simulink model "A1_MIM0_DigiTwin_4cm_JG_BM_2017b"  (R2017b)
settings: Solver=VariableStepAuto  StartTime=0.0  StopTime=tsim  RelTol=1e-3
InitFcn:
  | tsim=1000
  | sg=1;
  | Ts=500 %500% deseado 890-->Ts modelo
  | wn=5.8335/Ts; %2ord
  | wp=4/Ts; %np=1.5; 1ord
  | wt1=8*wn
  | wt=3.5*wn
  | wt3=3.49*wn
  | nf=2.5; %[1.2 1.5 1.75 2 2.5]
  | %Tfp=1/(np*wp)
  | Tf= 1/(nf*wn) % f del filtro;
  | nf3=5
  | Tf3= 1/(nf3*wn)
  | Rpc=0.09 % cold side resistor
  | Rph= 0.6 % hot side resistor
  | Tamb=273.15+15 % ambiental temp
  | Tin=273.15+15 % initial temp of mass
  | %TinA= 284.9405 % internal air Inicial temp
  | %TinAis=  294.0300 % initial Temp Mass insolat
  | %Tp1=283  %ideal temp of  peltier cells
  | %Tp2=Tp1
  | 
  | %Peltier Cells parameter
  | Th=323 % [K]
  | TinH=298
  | TinC=298 %
  | dTmax=75 % 70.5 [K]
  | Vmax= 16.4 % 13.9 [v]
  | Imax= 6.4 % 4  [A]
  | Rth= (dTmax/(Vmax*Imax))*(2*Th/(Th-dTmax)) % Termal Res [K/W]
  | am= Vmax/ Th %  0.054 Seebeck Coef []
  | ReC=Vmax*(Th-dTmax)/(Th*Imax) %range [1.6 1.96 2.5]
  | %Re= 2.3 %2.65   [2.6584  2.9592 3.26]  at 300 K
  | Mc=0.0135; %0.0045  Cool mass [kg]
  | Mh=0.0135; %0.0045
  | Cesp=1262  %1262.2 345
  | %TinL=300
  | %CespL=100 %45
  | %Mload=100%100-0.065 0.001
  | %Rload=1%5.5
  | 
  | 
  | % --Copper & aluminum plate
  | Da= 8960; %2700 [Kg/m^3] density
  | Qs= 390; %970 Specific heat [J/(Kg*K)]
  | Thi =0.00508; % 0.0033 Thickness [m]
  | L = 0.04; %0.03 length [m]
  | L1=0.035;
  | W=0.04; % 0.03 width  [m]
  | W1=0.01; W2=0.03;  W3=0.015;
  | Va= L*W*Thi % 2,97 E-6 [m^3] Dif of Volume
  | M=Da*Va % 0.00801 [kg]  % Al Dif of Mass
  | 
  | %--- Air Properties
  | Thi_air=0.015 % Thickness of air
  | Dair=1.29 % [Kg/m^3] density
  | Vair= L*W*Thi_air % E-6 [m^3] Dif of Volume
  | Mair=Dair*Vair %  [kg]  % Al Dif of Mass
  | 
  | % thermal conductivity [W/(m*K)]
  | K=401; %200  Aluminum
  | Km=11 % thermal paste. (between Al and peltier cell)
  | Ka=0.02 % air
  | % Natural Convection coefficient [W/(m^2*K)]
  | ha=75  % 5 <15<25 max
  | %  Forced Convection coefficient [W/(m^2*K)]
  | %ha=25  % 25< 138 <250
  | Thi_m= 0.001 % thermal paste Thickness
  | %Thermal Resistors [K/W]
  | Rs= Thi/(K*W*L); % -->0.016; Vertical Transfer Al
  | Rm= Thi_m/(Km*W*L); % -->0.101; Vertical Transfer Thermal Paste
  | R=W/(K*Thi*L); % -->0.49 & 1.51;  X & Y-->R=2*Rtdx serial conection
  | Rzcd=0.5*Thi/(K*W*L);%0.0040 & % correction R changed for Rzcd
  | Rzcd1=0.5*Thi/(K*W1*L);Rzcd2=0.5*Thi/(K*W2*L); Rzcd3=0.5*Thi/(K*W3*L);
  | 
  | % serie of two Rcd with diff VolumneElement
  | R1x=0.5*R+0.5*W1/(K*Thi*L); R2x=0.5*R+0.5*W2/(K*Thi*L);
  | R3x=0.5*R+0.5*W3/(K*Thi*L);
  | R1y=L/(K*Thi*W1); R2y=L/(K*Thi*W2); R3y=L/(K*Thi*W3);% R=2*Rtdy
  | 
  | Rzcv=1/(ha*W*L); % air resistor convection zDir (44<Ra< 222)
  | Rzcv1=1/(ha*W1*L); Rzcv2=1/(ha*W2*L); Rzcv3=1/(ha*W3*L);
  | Ra=(Rzcv+Rzcd)/2; % 250.004 CONVECTION + CONDUCTION Rzcv>>+Rzcd
  | Ra1=(Rzcv1)/2+Rzcd1; Ra2=(Rzcv2+Rzcd2)/2; Ra3=(Rzcv3+Rzcd3)/2;
  | 
  | Rxcv=1/(ha*L*Thi); % L=W Rycv RESISTOR CONVECTION xDir and YDir
  | Rycv1=1/(ha*W1*Thi); Rycv2=1/(ha*W2*Thi); Rycv3=1/(ha*W3*Thi);
  | Rp=0.5*R+Rxcv; % series conec 2 cond resist with diff VolumneElement
  | %Edge resistor conduction + convection efect
  | Rxp1=Rxcv+0.5*W1/(K*Thi*L); Rxp3=Rxcv+0.5*W3/(K*Thi*L);
  | Ryp1=Rycv1+0.5*L/(K*Thi*W1); Ryp2=Rycv2+0.5*L/(K*Thi*W2);
  | Ryp3=Rycv3+0.5*L/(K*Thi*W3);
  | 
  | 
  | 
  | %Número de Biot
  | % Lc= V/A = T
  | %Bi=ha*Thi/K % < 0.2  sys conc
  | 
  | % Polystyrene box
  | hao=15;
  | kpo=0.026;
  | %Vint=2000*Vair; %[m^3]  % interior volume
  | %Vout=28*19*7e-6;  %[m^3] % vol with external box dimension
  | %Vpo=Vout-Vint; % insulation material volume
  | Tpo=0.05; %[m] Thickness Poly
  | Apo_i= 24*15e-4+15*15*2e-4+15*24*2e-4; %[m^2]
  | Apo_o=34*25e-4+25*25*2e-4+25*34*2e-4;   %[m^2]
  | Vpo=Apo_i*Tpo
  | Dpo=33; % [km/m^3]
  | Mpo=Dpo*Vpo; % [kg]
  | 
  | %convection area without inferior face.
  | Rpo_i= Tpo/(kpo*Apo_i)% conduction resistor.
  | %Rpo_o= Tpo/(kpo*Apo_o)
  | Rao=1/(hao*Apo_o);  %  Convection resistor
  | Rai=1/(ha*Apo_i);
undefined symbols (not defined in the file or in its folder): TinA, TinAis, ymax, ymin
libraries: fl_lib x233, nesl_utility x61, simulink x6, ee_lib x4
(part 1 of 2)
settings Model: OrderedModelArguments=off  Creator=arca_  LastModifiedBy=jairo

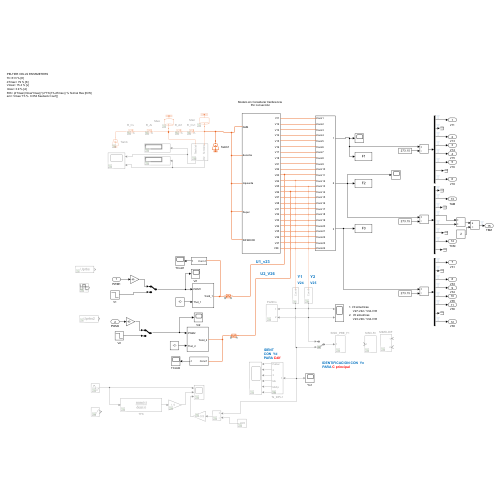
[thumbnail: Simulink's stored preview of the top-level diagram]
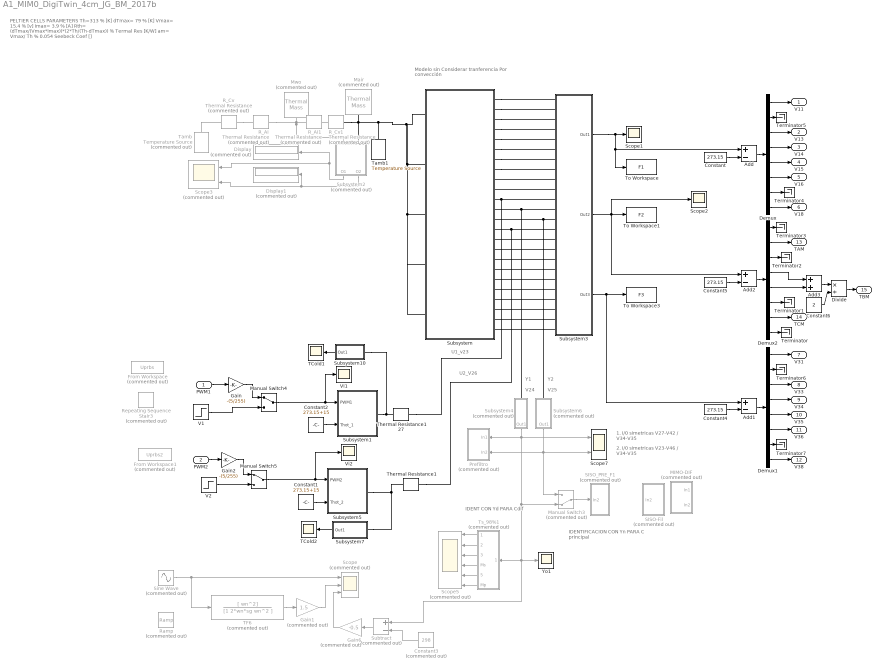
== system A1_MIM0_DigiTwin_4cm_JG_BM_2017b ==
  note: IDENT
      | CON Yd
      | PARA Cdif
  note: U1_v23
  note: 1. I/0 simetricas
      |      V27-V42 / V34-V35
  note: Modelo sin Considerar tranferencia
      | Por convección
  note: PELTIER CELLS PARAMETERS
      | Th=313 % [K]
      | dTmax= 79 % [K]
      | Vmax= 15.4 % [v]
      | Imax= 3.9 % [A]
      | Rth= (dTmax/(Vmax*Imax))*(2*Th/(Th-dTmax)) % Termal Res [K/W]
      | am= Vmax/ Th % 0.054 Seebeck Coef []
  note: 2.  I/0 simetricas
      |      V23-V46 / V34-V35
  note: U2_V26
  note: Y1
  note: Y2
  note: IDENTIFICACION CON Yn
      | PARA C principal
  note: V24
  note: V25
  PWM1 : Inport
  PWM2 : Inport  Port=2
  Add : Sum  Inputs=+-
  Add1 : Sum  Inputs=+-
  Add2 : Sum  Inputs=+-
  Add3 : Sum
  Constant : Constant  Value=273.15
  Constant1 : Constant  Value=273.15+15
  Constant2 : Constant  Value=273.15+15
  Constant3 : Constant  Commented=on  Value=298
  Constant4 : Constant  Value=273.15
  Constant5 : Constant  Value=273.15
  Constant6 : Constant  Value=2
  Demux : Demux  Outputs=8
  Demux1 : Demux  Outputs=8
  Demux2 : Demux  Outputs=8
  Display : Display  Commented=on
  Display1 : Display  Commented=on
  Divide : Product  Inputs=*/
  From Workspace : FromWorkspace  Commented=on  VariableName=Uprbs  SampleTime=1
  From Workspace1 : FromWorkspace  Commented=on  VariableName=Uprbs2  SampleTime=1
  Gain : Gain  Gain=-(5/255)
  Gain1 : Gain  Commented=on  Gain=1.5
  Gain2 : Gain  Gain=-(5/255)
  Gain6 : Gain  Commented=on  Gain=-0.5
  MIMO-DIF : Subsystem  Commented=on
  Mair : fl_lib/Thermal/Thermal Elements/Thermal Mass  Commented=on  mass=40*Mair kg  sp_heat=1000 J/kg/K  num_ports=foundation.enum.numPorts2.one  T_specify=on  T_priority=High  T=TinA K  T_nominal_specify=off  T_nominal_unit=K  T_nominal_value=1  Q_specify=off  Q_priority=None  Q=0 W  Q_nominal_specify=off  Q_nominal_unit=W  Q_nominal_value=1
  Manual Switch3 : ManualSwitch  Commented=on  CurrentSetting=0
  Manual Switch4 : ManualSwitch
  Manual Switch5 : ManualSwitch
  Mwo : fl_lib/Thermal/Thermal Elements/Thermal Mass  Commented=on  mass=Mpo kg  sp_heat=1200 J/kg/K  num_ports=foundation.enum.numPorts2.one  T_specify=on  T_priority=High  T=TinAis K  T_nominal_specify=off  T_nominal_unit=K  T_nominal_value=1  Q_specify=off  Q_priority=None  Q=0 W  Q_nominal_specify=off  Q_nominal_unit=W  Q_nominal_value=1
  Prefiltro : Subsystem  Commented=on
  R_Ai : fl_lib/Thermal/Thermal Elements/Thermal Resistance  Commented=on  resistance=Rpo_i/2 K/W  T_specify=off  T_priority=None  T=0 K  T_nominal_specify=off  T_nominal_unit=K  T_nominal_value=1  Q_specify=off  Q_priority=None  Q=0 W  Q_nominal_specify=off  Q_nominal_unit=W  Q_nominal_value=1
  R_Ai1 : fl_lib/Thermal/Thermal Elements/Thermal Resistance  Commented=on  resistance=Rpo_i/2 K/W  T_specify=off  T_priority=None  T=0 K  T_nominal_specify=off  T_nominal_unit=K  T_nominal_value=1  Q_specify=off  Q_priority=None  Q=0 W  Q_nominal_specify=off  Q_nominal_unit=W  Q_nominal_value=1
  R_Cv : fl_lib/Thermal/Thermal Elements/Thermal Resistance  Commented=on  resistance=Rao K/W  T_specify=off  T_priority=None  T=0 K  T_nominal_specify=off  T_nominal_unit=K  T_nominal_value=1  Q_specify=off  Q_priority=None  Q=0 W  Q_nominal_specify=off  Q_nominal_unit=W  Q_nominal_value=1
  R_Cv1 : fl_lib/Thermal/Thermal Elements/Thermal Resistance  Commented=on  resistance=Rai K/W  T_specify=off  T_priority=None  T=0 K  T_nominal_specify=off  T_nominal_unit=K  T_nominal_value=1  Q_specify=off  Q_priority=None  Q=0 W  Q_nominal_specify=off  Q_nominal_unit=W  Q_nominal_value=1
  Ramp : simulink/Sources/Ramp  Commented=on  slope=-44/1800  start=0  X0=0
  Repeating Sequence Stair3 : simulink/Sources/Repeating Sequence Stair  Commented=on  OutValues=[ -5 5 -5 ]'  tsamp=2000  OutMin=[]  OutMax=[]  OutDataTypeStr=float('double')  OutputDataTypeScalingMode=Specify via dialog  OutDataType=float('double')  ConRadixGroup=Best Precision: Vector-wise  OutScaling=2^-12
  SISO-Fil : Subsystem  Commented=on
  SISO_PRE_F1 : Subsystem  Commented=on
  Scope : Scope  Commented=on  NumInputPorts=3
  Scope1 : Scope
  Scope2 : Scope
  Scope3 : Scope  Commented=on  NumInputPorts=2
  Scope5 : Scope  Commented=on  NumInputPorts=6
  Scope7 : Scope  NumInputPorts=2
  Sine Wave : Sin  Commented=on  Amplitude=5  Frequency=0.007  SampleTime=0
  Subsystem : Subsystem
  Subsystem1 : Subsystem
  Subsystem10 : Subsystem
  Subsystem2 : Subsystem  Commented=on
  Subsystem3 : Subsystem
  Subsystem4 : Subsystem  Commented=on
  Subsystem5 : Subsystem
  Subsystem6 : Subsystem  Commented=on
  Subsystem7 : Subsystem
  Subtract : Sum  Commented=on  Inputs=+-
  TCold1 : Scope
  TCold2 : Scope
  TF6 : TransferFcn  Commented=on  Numerator=[ wn^2]  Denominator=[1 2*wn*sg wn^2 ]
  Tamb : fl_lib/Thermal/Thermal Sources/Temperature Source  Commented=on  temperature=Tamb K
  Tamb1 : fl_lib/Thermal/Thermal Sources/Temperature Source  temperature=Tamb K
  Terminator{,1..7} (8 alike) : Terminator
  Thermal Resistance1 : fl_lib/Thermal/Thermal Elements/Thermal Resistance  resistance=Rpc K/W  T_specify=off  T_priority=None  T=0 K  T_nominal_specify=off  T_nominal_unit=K  T_nominal_value=1  Q_specify=off  Q_priority=None  Q=0 W  Q_nominal_specify=off  Q_nominal_unit=W  Q_nominal_value=1
  Thermal Resistance127 : fl_lib/Thermal/Thermal Elements/Thermal Resistance  resistance=Rpc K/W  T_specify=off  T_priority=None  T=0 K  T_nominal_specify=off  T_nominal_unit=K  T_nominal_value=1  Q_specify=off  Q_priority=None  Q=0 W  Q_nominal_specify=off  Q_nominal_unit=W  Q_nominal_value=1
  To Workspace : ToWorkspace  VariableName=F1  SampleTime=-1
  To Workspace1 : ToWorkspace  VariableName=F2  SampleTime=-1
  To Workspace3 : ToWorkspace  VariableName=F3  SampleTime=-1
  Ts_98%1 : Subsystem  Commented=on
  V1 : Step  Time=0  After=-5  SampleTime=0
  V2 : Step  Time=0  After=-5  SampleTime=0
  Vi1 : Scope
  Vi2 : Scope
  Yo1 : Scope
  V11 : Outport
  V13 : Outport  Port=2
  V14 : Outport  Port=3
  V15 : Outport  Port=4
  V16 : Outport  Port=5
  V18 : Outport  Port=6
  V31 : Outport  Port=7
  V33 : Outport  Port=8
  V34 : Outport  Port=9
  V35 : Outport  Port=10
  V36 : Outport  Port=11
  V38 : Outport  Port=12
  TAM : Outport  Port=13
  TCM : Outport  Port=14
  TBM : Outport  Port=15
  wires:
  Subsystem2/1(O1) -> Scope3/1, Display/1
  Subsystem2/2(O2) -> Display1/1, Scope3/2
  Manual Switch5/1 -> Vi2/1, Subsystem5/1(PWM2)
  Manual Switch3/1 -> SISO_PRE_F1/1(In2)
  Subsystem6/1(Out1) -> Manual Switch3/1, Prefiltro/2(In2), Scope7/2
  Subsystem10/1(Out1) -> TCold1/1
  Constant2/1 -> Subsystem1/2(Thot_1)
  Manual Switch4/1 -> Vi1/1, Subsystem1/1(PWM1)
  Sine Wave/1 -> Scope/1, TF6/1
  V2/1 -> Manual Switch5/2
  Constant1/1 -> Subsystem5/2(Thot_2)
  Subsystem7/1(Out1) -> TCold2/1
  Ts_98%1/3(Out3) -> Scope5/3
  Ts_98%1/1(Peltier) -> Scope5/1
  Ts_98%1/2(Out2) -> Scope5/2
  Ts_98%1/5(MsFp) -> Scope5/5
  Ts_98%1/6(Mp) -> Scope5/6
  Subsystem4/1(Out1) -> Subtract/1, Ts_98%1/1(In1), Yo1/1, Manual Switch3/2, Prefiltro/1(In1), Scope7/1
  Ts_98%1/4(Ms) -> Scope5/4
  Subtract/1 -> Gain6/1
  Constant3/1 -> Subtract/2
  Gain6/1 -> Scope/3
  TF6/1 -> Gain1/1
  Gain1/1 -> Scope/2
  V1/1 -> Manual Switch4/2
  Gain/1 -> Manual Switch4/1
  Gain2/1 -> Manual Switch5/1
  PWM1/1 -> Gain/1
  PWM2/1 -> Gain2/1
  Constant/1 -> Add/2
  Subsystem3/1(Out1) -> Add/1, To Workspace/1, Scope1/1
  Add/1 -> Demux/1
  Demux/1 -> V11/1
  Demux/3 -> V13/1
  Demux/4 -> V14/1
  Demux/5 -> V15/1
  Demux/6 -> V16/1
  Demux/8 -> V18/1
  Demux1/4 -> V34/1
  Demux1/3 -> V33/1
  Subsystem3/3(Out3) -> Add1/1, To Workspace3/1
  Demux1/6 -> V36/1
  Add1/1 -> Demux1/1
  Demux1/1 -> V31/1
  Constant4/1 -> Add1/2
  Demux1/5 -> V35/1
  Demux1/8 -> V38/1
  Constant5/1 -> Add2/2
  Subsystem3/2(Out2) -> Add2/1, Scope2/1, To Workspace1/1
  Add2/1 -> Demux2/1
  Demux2/2 -> TAM/1
  Demux2/7 -> TCM/1
  Add3/1 -> Divide/1
  Demux2/4 -> Add3/1
  Demux2/5 -> Add3/2
  Constant6/1 -> Divide/2
  Divide/1 -> TBM/1
  Demux2/8 -> Terminator/1
  Demux2/6 -> Terminator1/1
  Demux2/3 -> Terminator2/1
  Demux2/1 -> Terminator3/1
  Demux/7 -> Terminator4/1
  Demux/2 -> Terminator5/1
  Demux1/2 -> Terminator6/1
  Demux1/7 -> Terminator7/1
  connections:
  Mair/LConn1 -- Subsystem/LConn5 -- Subsystem/LConn4 -- Subsystem/LConn3 -- Subsystem/LConn2 -- Subsystem/LConn1 -- Tamb1/LConn1 -- Subsystem2/LConn2 -- R_Cv1/LConn1
  R_Cv/RConn1 -- Tamb/LConn1
  Mwo/LConn1 -- Subsystem2/LConn1 -- R_Ai/LConn1 -- R_Ai1/RConn1
  R_Cv/LConn1 -- R_Ai/RConn1
  R_Cv1/RConn1 -- R_Ai1/LConn1
  Subsystem1/RConn1 -- Subsystem10/LConn1 -- Thermal Resistance127/RConn1
  Subsystem7/LConn1 -- Subsystem5/RConn1 -- Thermal Resistance1/RConn1
  Subsystem/RConn1 -- Subsystem3/LConn1
  Subsystem/RConn2 -- Subsystem3/LConn2
  Subsystem/RConn3 -- Subsystem3/LConn3
  Subsystem/RConn4 -- Subsystem3/LConn4
  Subsystem/RConn5 -- Subsystem3/LConn5
  Subsystem/RConn6 -- Subsystem3/LConn6
  Subsystem/RConn7 -- Subsystem3/LConn7
  Subsystem/RConn8 -- Subsystem3/LConn8
  Subsystem3/LConn9 -- Subsystem/RConn9
  Subsystem3/LConn10 -- Subsystem/RConn10
  Subsystem3/LConn12 -- Subsystem4/LConn1 -- Subsystem/RConn12
  Subsystem3/LConn11 -- Thermal Resistance127/LConn1 -- Subsystem/RConn11
  Subsystem3/LConn13 -- Subsystem6/LConn1 -- Subsystem/RConn13
  Subsystem3/LConn14 -- Thermal Resistance1/LConn1 -- Subsystem/RConn14
  Subsystem3/LConn15 -- Subsystem/RConn15
  Subsystem3/LConn16 -- Subsystem/RConn16
  Subsystem3/LConn17 -- Subsystem/RConn17
  Subsystem3/LConn18 -- Subsystem/RConn18
  Subsystem3/LConn19 -- Subsystem/RConn19
  Subsystem3/LConn20 -- Subsystem/RConn20
  Subsystem3/LConn21 -- Subsystem/RConn21
  Subsystem3/LConn22 -- Subsystem/RConn22
  Subsystem3/LConn23 -- Subsystem/RConn23
  Subsystem3/LConn24 -- Subsystem/RConn24

== system A1_MIM0_DigiTwin_4cm_JG_BM_2017b/MIMO-DIF ==
  note: DE LAZO CERRADO CON FILTRO
      | A LAZO ABIERTO
  note: LAZO ABIERTO CON FILTRO
  In1 : Inport
  In2 : Inport  Port=2
  (Yr-Uv1-Uv2)Ol : Scope  NumInputPorts=3
  (Yr-Uv1-Uv2)cl : Scope  NumInputPorts=3
  Add1 : Sum
  Add3 : Sum  Inputs=+-
  Add4 : Sum  Inputs=++-
  Add5 : Sum  Commented=on  Inputs=+-
  Constant4 : Constant  Commented=on  Value=298
  Derivative{1..2,8..9} (4 alike) : Derivative
  Gain1 : Gain  Gain=1/nf
  Gain10 : Gain  Gain=2
  Gain{4..5,9,11} (4 alike) : Gain  Gain=1/wn
  Gain3 : Gain  Gain=2
  ToDif : Scope
  Transfer Fcn1 : TransferFcn  Denominator=[Tf 1]
  Transfer Fcn2 : TransferFcn  Denominator=[Tf 1]
  Transfer Fcn3 : TransferFcn  Numerator=[1 2*wn 0]  Denominator=[wn^2*Tf^2 2*wn^2*Tf wn^2]
  Transfer Fcn6 : TransferFcn  Numerator=[(nf^2-1) 2*wn*nf*(nf-1) 0]  Denominator=[1 2*nf*wn nf^2*wn^2]
  Uv{1..4} (4 alike) : Scope
  wires:
  Gain9/1 -> Derivative8/1
  Derivative9/1 -> Gain11/1
  Transfer Fcn6/1 -> (Yr-Uv1-Uv2)cl/3, Uv2/1
  Derivative8/1 -> Add4/1
  Transfer Fcn1/1 -> Uv3/1, (Yr-Uv1-Uv2)Ol/2
  Gain11/1 -> Gain1/1, Gain10/1, Gain9/1
  Transfer Fcn3/1 -> Uv4/1, (Yr-Uv1-Uv2)Ol/3
  Derivative2/1 -> Gain4/1
  Add1/1 -> Transfer Fcn1/1
  Gain3/1 -> Add1/2
  Gain10/1 -> Add4/2
  Gain1/1 -> Add4/3
  Transfer Fcn2/1 -> (Yr-Uv1-Uv2)cl/2, Uv1/1
  Gain5/1 -> Derivative1/1
  Gain4/1 -> Gain5/1, Gain3/1
  Add4/1 -> Transfer Fcn2/1
  Derivative1/1 -> Add1/1
  Add3/1 -> Transfer Fcn3/1, (Yr-Uv1-Uv2)Ol/1, Derivative2/1, Transfer Fcn6/1, Derivative9/1, (Yr-Uv1-Uv2)cl/1, ToDif/1
  In2/1 -> Add3/1
  In1/1 -> Add3/2
  Constant4/1 -> Add5/2
  ? -> Add5/1

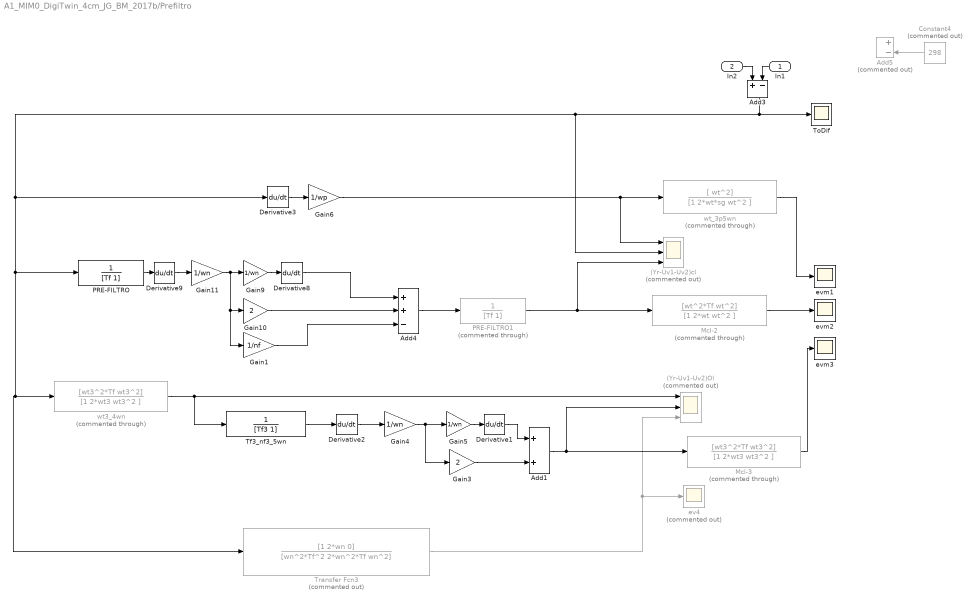
== system A1_MIM0_DigiTwin_4cm_JG_BM_2017b/Prefiltro ==
  In1 : Inport
  In2 : Inport  Port=2
  (Yr-Uv1-Uv2)Ol : Scope  Commented=on  NumInputPorts=3
  (Yr-Uv1-Uv2)cl : Scope  Commented=on  NumInputPorts=3
  Add1 : Sum
  Add3 : Sum  Inputs=+-
  Add4 : Sum  Inputs=++-
  Add5 : Sum  Commented=on  Inputs=+-
  Constant4 : Constant  Commented=on  Value=298
  Derivative{1..3,8..9} (5 alike) : Derivative
  Gain1 : Gain  Gain=1/nf
  Gain10 : Gain  Gain=2
  Gain{4..5,9,11} (4 alike) : Gain  Gain=1/wn
  Gain3 : Gain  Gain=2
  Gain6 : Gain  Gain=1/wp
  Mcl-2 : TransferFcn  Commented=through  Numerator=[wt^2*Tf wt^2]  Denominator=[1 2*wt wt^2 ]
  Mcl-3 : TransferFcn  Commented=through  Numerator=[wt3^2*Tf wt3^2]  Denominator=[1 2*wt3 wt3^2 ]
  PRE-FILTRO : TransferFcn  Denominator=[Tf 1]
  PRE-FILTRO1 : TransferFcn  Commented=through  Denominator=[Tf 1]
  Tf3_nf3_5wn : TransferFcn  Denominator=[Tf3 1]
  ToDif : Scope
  Transfer Fcn3 : TransferFcn  Commented=on  Numerator=[1 2*wn 0]  Denominator=[wn^2*Tf^2 2*wn^2*Tf wn^2]
  ev4 : Scope  Commented=on
  evm1 : Scope
  evm2 : Scope
  evm3 : Scope
  wt3_4wn : TransferFcn  Commented=through  Numerator=[wt3^2*Tf wt3^2]  Denominator=[1 2*wt3 wt3^2 ]
  wt_3p5wn : TransferFcn  Commented=through  Numerator=[ wt^2]  Denominator=[1 2*wt*sg wt^2 ]
  wires:
  In2/1 -> Add3/1
  In1/1 -> Add3/2
  Constant4/1 -> Add5/2
  ? -> Add5/1
  Gain9/1 -> Derivative8/1
  Gain3/1 -> Add1/2
  Derivative9/1 -> Gain11/1
  Derivative3/1 -> Gain6/1
  Add3/1 -> (Yr-Uv1-Uv2)cl/2, PRE-FILTRO/1, Transfer Fcn3/1, wt3_4wn/1, Derivative3/1, ToDif/1
  Derivative8/1 -> Add4/1
  Mcl-2/1 -> evm2/1
  Gain4/1 -> Gain5/1, Gain3/1
  Mcl-3/1 -> evm3/1
  wt3_4wn/1 -> (Yr-Uv1-Uv2)Ol/1, Tf3_nf3_5wn/1
  Derivative1/1 -> Add1/1
  Gain1/1 -> Add4/3
  Gain10/1 -> Add4/2
  Derivative2/1 -> Gain4/1
  PRE-FILTRO/1 -> Derivative9/1
  Add4/1 -> PRE-FILTRO1/1
  wt_3p5wn/1 -> evm1/1
  Transfer Fcn3/1 -> ev4/1, (Yr-Uv1-Uv2)Ol/3
  Tf3_nf3_5wn/1 -> Derivative2/1
  Add1/1 -> (Yr-Uv1-Uv2)Ol/2, Mcl-3/1
  Gain5/1 -> Derivative1/1
  PRE-FILTRO1/1 -> (Yr-Uv1-Uv2)cl/3, Mcl-2/1
  Gain11/1 -> Gain9/1, Gain10/1, Gain1/1
  Gain6/1 -> (Yr-Uv1-Uv2)cl/1, wt_3p5wn/1

== system A1_MIM0_DigiTwin_4cm_JG_BM_2017b/SISO-Fil ==
  note: LAZO ABIERTO CON FILTRO
  note: DE LAZO CERRADO CON FILTRO
      | A LAZO ABIERTO
  In2 : Inport
  (Yr-Uv1-Uv2)Ol : Scope  NumInputPorts=3
  (Yr-Uv1-Uv2)cl : Scope  NumInputPorts=3
  Add1 : Sum
  Add3 : Sum  Inputs=+-
  Add4 : Sum  Inputs=++-
  Constant4 : Constant  Commented=on  Value=298
  Derivative{1..2,8..9} (4 alike) : Derivative
  Gain1 : Gain  Gain=1/nf
  Gain10 : Gain  Gain=2
  Gain{4..5,9,11} (4 alike) : Gain  Gain=1/wn
  Gain3 : Gain  Gain=2
  ToDif : Scope
  Transfer Fcn1 : TransferFcn  Denominator=[Tf 1]
  Transfer Fcn2 : TransferFcn  Denominator=[Tf 1]
  Transfer Fcn3 : TransferFcn  Numerator=[1 2*wn 0]  Denominator=[wn^2*Tf^2 2*wn^2*Tf wn^2]
  Transfer Fcn6 : TransferFcn  Numerator=[(nf^2-1) 2*wn*nf*(nf-1) 0]  Denominator=[1 2*nf*wn nf^2*wn^2]
  Uv{1..4} (4 alike) : Scope
  wires:
  Constant4/1 -> Add3/2
  In2/1 -> Add3/1
  Add3/1 -> ToDif/1, (Yr-Uv1-Uv2)cl/1, Derivative9/1, Transfer Fcn6/1, Derivative2/1, (Yr-Uv1-Uv2)Ol/1, Transfer Fcn3/1
  Derivative1/1 -> Add1/1
  Add4/1 -> Transfer Fcn2/1
  Gain4/1 -> Gain3/1, Gain5/1
  Gain5/1 -> Derivative1/1
  Transfer Fcn2/1 -> Uv1/1, (Yr-Uv1-Uv2)cl/2
  Gain1/1 -> Add4/3
  Gain10/1 -> Add4/2
  Gain3/1 -> Add1/2
  Add1/1 -> Transfer Fcn1/1
  Derivative2/1 -> Gain4/1
  Transfer Fcn3/1 -> (Yr-Uv1-Uv2)Ol/3, Uv4/1
  Gain11/1 -> Gain9/1, Gain10/1, Gain1/1
  Transfer Fcn1/1 -> (Yr-Uv1-Uv2)Ol/2, Uv3/1
  Derivative8/1 -> Add4/1
  Transfer Fcn6/1 -> Uv2/1, (Yr-Uv1-Uv2)cl/3
  Derivative9/1 -> Gain11/1
  Gain9/1 -> Derivative8/1

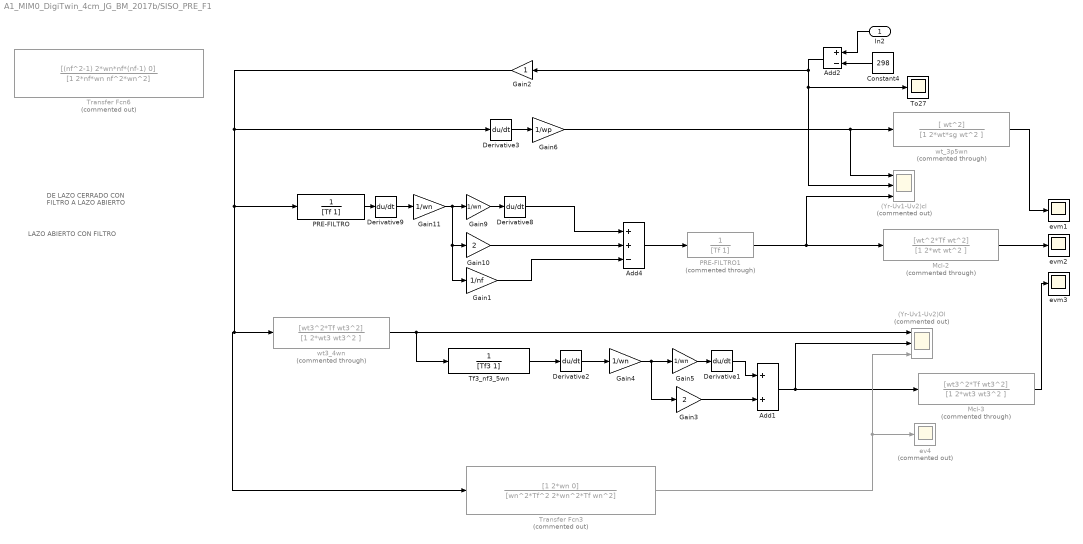
== system A1_MIM0_DigiTwin_4cm_JG_BM_2017b/SISO_PRE_F1 ==
  note: LAZO ABIERTO CON FILTRO
  note: DE LAZO CERRADO CON FILTRO
      | A LAZO ABIERTO
  In2 : Inport
  (Yr-Uv1-Uv2)Ol : Scope  Commented=on  NumInputPorts=3
  (Yr-Uv1-Uv2)cl : Scope  Commented=on  NumInputPorts=3
  Add1 : Sum
  Add2 : Sum  Inputs=+-
  Add4 : Sum  Inputs=++-
  Constant4 : Constant  Value=298
  Derivative{1..3,8..9} (5 alike) : Derivative
  Gain1 : Gain  Gain=1/nf
  Gain10 : Gain  Gain=2
  Gain{4..5,9,11} (4 alike) : Gain  Gain=1/wn
  Gain2 : Gain
  Gain3 : Gain  Gain=2
  Gain6 : Gain  Gain=1/wp
  Mcl-2 : TransferFcn  Commented=through  Numerator=[wt^2*Tf wt^2]  Denominator=[1 2*wt wt^2 ]
  Mcl-3 : TransferFcn  Commented=through  Numerator=[wt3^2*Tf wt3^2]  Denominator=[1 2*wt3 wt3^2 ]
  PRE-FILTRO : TransferFcn  Denominator=[Tf 1]
  PRE-FILTRO1 : TransferFcn  Commented=through  Denominator=[Tf 1]
  Tf3_nf3_5wn : TransferFcn  Denominator=[Tf3 1]
  To27 : Scope
  Transfer Fcn3 : TransferFcn  Commented=on  Numerator=[1 2*wn 0]  Denominator=[wn^2*Tf^2 2*wn^2*Tf wn^2]
  Transfer Fcn6 : TransferFcn  Commented=on  Numerator=[(nf^2-1) 2*wn*nf*(nf-1) 0]  Denominator=[1 2*nf*wn nf^2*wn^2]
  ev4 : Scope  Commented=on
  evm1 : Scope
  evm2 : Scope
  evm3 : Scope
  wt3_4wn : TransferFcn  Commented=through  Numerator=[wt3^2*Tf wt3^2]  Denominator=[1 2*wt3 wt3^2 ]
  wt_3p5wn : TransferFcn  Commented=through  Numerator=[ wt^2]  Denominator=[1 2*wt*sg wt^2 ]
  wires:
  Gain2/1 -> PRE-FILTRO/1, Transfer Fcn3/1, wt3_4wn/1, Derivative3/1
  Gain3/1 -> Add1/2
  Add1/1 -> (Yr-Uv1-Uv2)Ol/2, Mcl-3/1
  Gain4/1 -> Gain5/1, Gain3/1
  Derivative1/1 -> Add1/1
  Gain5/1 -> Derivative1/1
  Add2/1 -> (Yr-Uv1-Uv2)cl/2, To27/1, Gain2/1
  Transfer Fcn3/1 -> ev4/1, (Yr-Uv1-Uv2)Ol/3
  Derivative2/1 -> Gain4/1
  Gain1/1 -> Add4/3
  In2/1 -> Add2/1
  Gain10/1 -> Add4/2
  Gain11/1 -> Gain9/1, Gain10/1, Gain1/1
  Derivative8/1 -> Add4/1
  Constant4/1 -> Add2/2
  Gain9/1 -> Derivative8/1
  Gain6/1 -> (Yr-Uv1-Uv2)cl/1, wt_3p5wn/1
  PRE-FILTRO/1 -> Derivative9/1
  Tf3_nf3_5wn/1 -> Derivative2/1
  Derivative9/1 -> Gain11/1
  Add4/1 -> PRE-FILTRO1/1
  Derivative3/1 -> Gain6/1
  Mcl-3/1 -> evm3/1
  PRE-FILTRO1/1 -> (Yr-Uv1-Uv2)cl/3, Mcl-2/1
  wt_3p5wn/1 -> evm1/1
  wt3_4wn/1 -> (Yr-Uv1-Uv2)Ol/1, Tf3_nf3_5wn/1
  Mcl-2/1 -> evm2/1

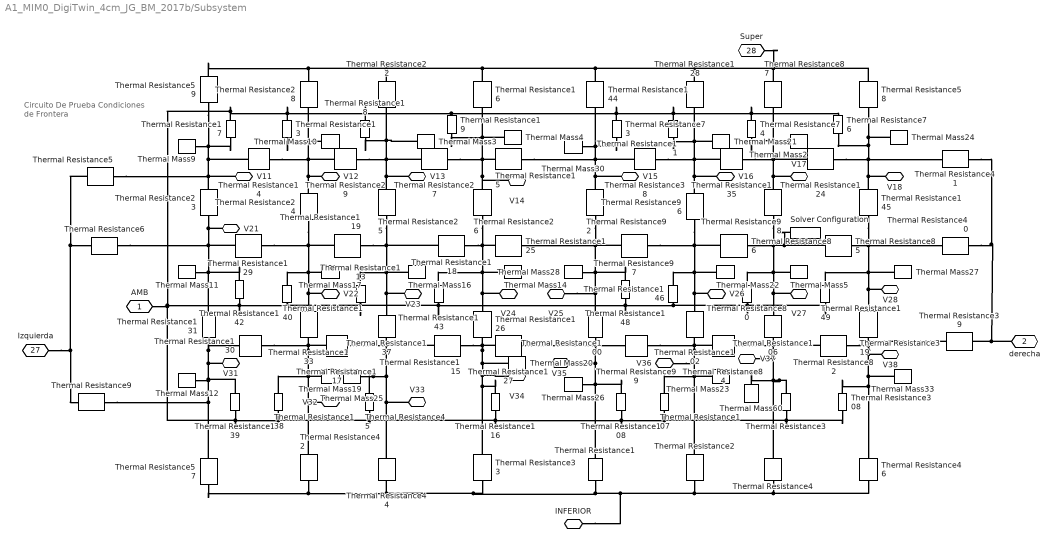
== system A1_MIM0_DigiTwin_4cm_JG_BM_2017b/Subsystem ==
  note: Circuito De Prueba
      | Condiciones de Frontera
  Solver Configuration : nesl_utility/Solver Configuration  PhysicalDomain=network_engine_domain  SubClassName=solver  LeftPortType=input  RightPortType=generic  Tones=[]  Harmonics=[]  SimulateNoise=off  Profile=off  UseLocalSampling=off  EnableSwitchedLinearOptims=on  FrequencyDomain=off  UseCCode=off  RelTol=0.001  AbsTol=1e-06  MinStep=1e-09  ToWorkspace=off  RevertToSquareIcSolve=off  NumHomotopyIterations=100  PhasorMode=off  PhasorModeNumHarmonics=1  ConsistencySolver=NEWTON_FTOL  IndexReductionMethod=DerivativeReplacement  DoDC=off  ResidualTolerance=1e-09  ConsistencyTolSource=GLOBAL  ConsistencyAbsTol=0.001  ConsistencyRelTol=0.001  ConsistencyTolFactor=0.001  UseLocalSolver=off  LocalSolverChoice=NE_BACKWARD_EULER_ADVANCER  ResolveIndetEquations=on  FunctionEvalNumThread=1  LocalSolverSampleTime=0.001  DoFixedCost=off  MaxNonlinIter=3  MaxModeIter=2  ComputeImpulses=off  ImpulseIterations=2  LinearAlgebra=Sparse  LinearAlgebraNumThread=0  EquationFormulation=NE_TIME_EF  DelaysMemoryBudget=1024  AutomaticFiltering=on  FilteringTimeConstant=0.001  PartitionStorageMethod=AS_NEEDED  PartitionMemoryBudget=1024  PartitionMethod=FAST
  Thermal Mass{2..5,9..12,14,16..17,19..28,30,33,60} (24 alike) : fl_lib/Thermal/Thermal Elements/Thermal Mass  mass=M kg  sp_heat=Qs J/kg/K  num_ports=foundation.enum.numPorts2.one  T_specify=on  T_priority=High  T=Tin K  T_nominal_specify=off  T_nominal_unit=K  T_nominal_value=1  Q_specify=off  Q_priority=None  Q=0 W  Q_nominal_specify=off  Q_nominal_unit=W  Q_nominal_value=1
  Thermal Resistance1 : fl_lib/Thermal/Thermal Elements/Thermal Resistance  resistance=Ryp2 K/W  T_specify=off  T_priority=None  T=0 K  T_nominal_specify=off  T_nominal_unit=K  T_nominal_value=1  Q_specify=off  Q_priority=None  Q=0 W  Q_nominal_specify=off  Q_nominal_unit=W  Q_nominal_value=1
  Thermal Resistance{24..27,29,82,84..86,92,96,98,100,102,106,115,117..119,124,126,133,135,137,145,319} (26 alike) : fl_lib/Thermal/Thermal Elements/Thermal Resistance  resistance=R K/W  T_specify=off  T_priority=None  T=0 K  T_nominal_specify=off  T_nominal_unit=K  T_nominal_value=1  Q_specify=off  Q_priority=None  Q=0 W  Q_nominal_specify=off  Q_nominal_unit=W  Q_nominal_value=1
  Thermal Resistance{3,11,13,18..19,45,74,80,107,116,138,140,143} (13 alike) : fl_lib/Thermal/Thermal Elements/Thermal Resistance  resistance=Ra K/W  T_specify=off  T_priority=None  T=0 K  T_nominal_specify=off  T_nominal_unit=K  T_nominal_value=1  Q_specify=off  Q_priority=None  Q=0 W  Q_nominal_specify=off  Q_nominal_unit=W  Q_nominal_value=1
  Thermal Resistance108 : fl_lib/Thermal/Thermal Elements/Thermal Resistance  resistance=Ra2 K/W  T_specify=off  T_priority=None  T=0 K  T_nominal_specify=off  T_nominal_unit=K  T_nominal_value=1  Q_specify=off  Q_priority=None  Q=0 W  Q_nominal_specify=off  Q_nominal_unit=W  Q_nominal_value=1
  Thermal Resistance113 : fl_lib/Thermal/Thermal Elements/Thermal Resistance  resistance=2*Ra K/W  T_specify=off  T_priority=None  T=0 K  T_nominal_specify=off  T_nominal_unit=K  T_nominal_value=1  Q_specify=off  Q_priority=None  Q=0 W  Q_nominal_specify=off  Q_nominal_unit=W  Q_nominal_value=1
  Thermal Resistance{15,38,97,99,125,127} (6 alike) : fl_lib/Thermal/Thermal Elements/Thermal Resistance  resistance=R2x K/W  T_specify=off  T_priority=None  T=0 K  T_nominal_specify=off  T_nominal_unit=K  T_nominal_value=1  Q_specify=off  Q_priority=None  Q=0 W  Q_nominal_specify=off  Q_nominal_unit=W  Q_nominal_value=1
  Thermal Resistance{2,4,16,22,28,33,42,44,87,128} (10 alike) : fl_lib/Thermal/Thermal Elements/Thermal Resistance  resistance=Rp K/W  T_specify=off  T_priority=None  T=0 K  T_nominal_specify=off  T_nominal_unit=K  T_nominal_value=1  Q_specify=off  Q_priority=None  Q=0 W  Q_nominal_specify=off  Q_nominal_unit=W  Q_nominal_value=1
  Thermal Resistance129 : fl_lib/Thermal/Thermal Elements/Thermal Resistance  resistance=R1x K/W  T_specify=off  T_priority=None  T=0 K  T_nominal_specify=off  T_nominal_unit=K  T_nominal_value=1  Q_specify=off  Q_priority=None  Q=0 W  Q_nominal_specify=off  Q_nominal_unit=W  Q_nominal_value=1
  Thermal Resistance130 : fl_lib/Thermal/Thermal Elements/Thermal Resistance  resistance=R1x K/W  T_specify=off  T_priority=None  T=0 K  T_nominal_specify=off  T_nominal_unit=K  T_nominal_value=1  Q_specify=off  Q_priority=None  Q=0 W  Q_nominal_specify=off  Q_nominal_unit=W  Q_nominal_value=1
  Thermal Resistance131 : fl_lib/Thermal/Thermal Elements/Thermal Resistance  resistance=R1y K/W  T_specify=off  T_priority=None  T=0 K  T_nominal_specify=off  T_nominal_unit=K  T_nominal_value=1  Q_specify=off  Q_priority=None  Q=0 W  Q_nominal_specify=off  Q_nominal_unit=W  Q_nominal_value=1
  Thermal Resistance139 : fl_lib/Thermal/Thermal Elements/Thermal Resistance  resistance=Ra1 K/W  T_specify=off  T_priority=None  T=0 K  T_nominal_specify=off  T_nominal_unit=K  T_nominal_value=1  Q_specify=off  Q_priority=None  Q=0 W  Q_nominal_specify=off  Q_nominal_unit=W  Q_nominal_value=1
  Thermal Resistance14 : fl_lib/Thermal/Thermal Elements/Thermal Resistance  resistance=R1x K/W  T_specify=off  T_priority=None  T=0 K  T_nominal_specify=off  T_nominal_unit=K  T_nominal_value=1  Q_specify=off  Q_priority=None  Q=0 W  Q_nominal_specify=off  Q_nominal_unit=W  Q_nominal_value=1
  Thermal Resistance142 : fl_lib/Thermal/Thermal Elements/Thermal Resistance  resistance=Ra1 K/W  T_specify=off  T_priority=None  T=0 K  T_nominal_specify=off  T_nominal_unit=K  T_nominal_value=1  Q_specify=off  Q_priority=None  Q=0 W  Q_nominal_specify=off  Q_nominal_unit=W  Q_nominal_value=1
  Thermal Resistance144 : fl_lib/Thermal/Thermal Elements/Thermal Resistance  resistance=Ryp2 K/W  T_specify=off  T_priority=None  T=0 K  T_nominal_specify=off  T_nominal_unit=K  T_nominal_value=1  Q_specify=off  Q_priority=None  Q=0 W  Q_nominal_specify=off  Q_nominal_unit=W  Q_nominal_value=1
  Thermal Resistance146 : fl_lib/Thermal/Thermal Elements/Thermal Resistance  resistance=2*Ra K/W  T_specify=off  T_priority=None  T=0 K  T_nominal_specify=off  T_nominal_unit=K  T_nominal_value=1  Q_specify=off  Q_priority=None  Q=0 W  Q_nominal_specify=off  Q_nominal_unit=W  Q_nominal_value=1
  Thermal Resistance148 : fl_lib/Thermal/Thermal Elements/Thermal Resistance  resistance=Ra2 K/W  T_specify=off  T_priority=None  T=0 K  T_nominal_specify=off  T_nominal_unit=K  T_nominal_value=1  Q_specify=off  Q_priority=None  Q=0 W  Q_nominal_specify=off  Q_nominal_unit=W  Q_nominal_value=1
  Thermal Resistance149 : fl_lib/Thermal/Thermal Elements/Thermal Resistance  resistance=Ra3 K/W  T_specify=off  T_priority=None  T=0 K  T_nominal_specify=off  T_nominal_unit=K  T_nominal_value=1  Q_specify=off  Q_priority=None  Q=0 W  Q_nominal_specify=off  Q_nominal_unit=W  Q_nominal_value=1
  Thermal Resistance17 : fl_lib/Thermal/Thermal Elements/Thermal Resistance  resistance=Ra1 K/W  T_specify=off  T_priority=None  T=0 K  T_nominal_specify=off  T_nominal_unit=K  T_nominal_value=1  Q_specify=off  Q_priority=None  Q=0 W  Q_nominal_specify=off  Q_nominal_unit=W  Q_nominal_value=1
  Thermal Resistance23 : fl_lib/Thermal/Thermal Elements/Thermal Resistance  resistance=R1y K/W  T_specify=off  T_priority=None  T=0 K  T_nominal_specify=off  T_nominal_unit=K  T_nominal_value=1  Q_specify=off  Q_priority=None  Q=0 W  Q_nominal_specify=off  Q_nominal_unit=W  Q_nominal_value=1
  Thermal Resistance308 : fl_lib/Thermal/Thermal Elements/Thermal Resistance  resistance=Ra3 K/W  T_specify=off  T_priority=None  T=0 K  T_nominal_specify=off  T_nominal_unit=K  T_nominal_value=1  Q_specify=off  Q_priority=None  Q=0 W  Q_nominal_specify=off  Q_nominal_unit=W  Q_nominal_value=1
  Thermal Resistance{39..41,46,58} (5 alike) : fl_lib/Thermal/Thermal Elements/Thermal Resistance  resistance=Ryp3 K/W  T_specify=off  T_priority=None  T=0 K  T_nominal_specify=off  T_nominal_unit=K  T_nominal_value=1  Q_specify=off  Q_priority=None  Q=0 W  Q_nominal_specify=off  Q_nominal_unit=W  Q_nominal_value=1
  Thermal Resistance5 : fl_lib/Thermal/Thermal Elements/Thermal Resistance  resistance=Rxp1 K/W  T_specify=off  T_priority=None  T=0 K  T_nominal_specify=off  T_nominal_unit=K  T_nominal_value=1  Q_specify=off  Q_priority=None  Q=0 W  Q_nominal_specify=off  Q_nominal_unit=W  Q_nominal_value=1
  Thermal Resistance57 : fl_lib/Thermal/Thermal Elements/Thermal Resistance  resistance=Ryp1 K/W  T_specify=off  T_priority=None  T=0 K  T_nominal_specify=off  T_nominal_unit=K  T_nominal_value=1  Q_specify=off  Q_priority=None  Q=0 W  Q_nominal_specify=off  Q_nominal_unit=W  Q_nominal_value=1
  Thermal Resistance59 : fl_lib/Thermal/Thermal Elements/Thermal Resistance  resistance=Ryp1 K/W  T_specify=off  T_priority=None  T=0 K  T_nominal_specify=off  T_nominal_unit=K  T_nominal_value=1  Q_specify=off  Q_priority=None  Q=0 W  Q_nominal_specify=off  Q_nominal_unit=W  Q_nominal_value=1
  Thermal Resistance6 : fl_lib/Thermal/Thermal Elements/Thermal Resistance  resistance=Rxp1 K/W  T_specify=off  T_priority=None  T=0 K  T_nominal_specify=off  T_nominal_unit=K  T_nominal_value=1  Q_specify=off  Q_priority=None  Q=0 W  Q_nominal_specify=off  Q_nominal_unit=W  Q_nominal_value=1
  Thermal Resistance73 : fl_lib/Thermal/Thermal Elements/Thermal Resistance  resistance=Ra2 K/W  T_specify=off  T_priority=None  T=0 K  T_nominal_specify=off  T_nominal_unit=K  T_nominal_value=1  Q_specify=off  Q_priority=None  Q=0 W  Q_nominal_specify=off  Q_nominal_unit=W  Q_nominal_value=1
  Thermal Resistance76 : fl_lib/Thermal/Thermal Elements/Thermal Resistance  resistance=Ra3 K/W  T_specify=off  T_priority=None  T=0 K  T_nominal_specify=off  T_nominal_unit=K  T_nominal_value=1  Q_specify=off  Q_priority=None  Q=0 W  Q_nominal_specify=off  Q_nominal_unit=W  Q_nominal_value=1
  Thermal Resistance9 : fl_lib/Thermal/Thermal Elements/Thermal Resistance  resistance=Rxp1 K/W  T_specify=off  T_priority=None  T=0 K  T_nominal_specify=off  T_nominal_unit=K  T_nominal_value=1  Q_specify=off  Q_priority=None  Q=0 W  Q_nominal_specify=off  Q_nominal_unit=W  Q_nominal_value=1
  AMB : PMIOPort  Side=Left
  derecha : PMIOPort  Port=2  Side=Left
  V11 : PMIOPort  Port=3  Side=Right
  V12 : PMIOPort  Port=4  Side=Right
  V13 : PMIOPort  Port=5  Side=Right
  V14 : PMIOPort  Port=6  Side=Right
  V15 : PMIOPort  Port=7  Side=Right
  V16 : PMIOPort  Port=8  Side=Right
  V17 : PMIOPort  Port=9  Side=Right
  V18 : PMIOPort  Port=10  Side=Right
  V21 : PMIOPort  Port=11  Side=Right
  V22 : PMIOPort  Port=12  Side=Right
  V23 : PMIOPort  Port=13  Side=Right
  V24 : PMIOPort  Port=14  Side=Right
  V25 : PMIOPort  Port=15  Side=Right
  V26 : PMIOPort  Port=16  Side=Right
  V27 : PMIOPort  Port=17  Side=Right
  V28 : PMIOPort  Port=18  Side=Right
  V31 : PMIOPort  Port=19  Side=Right
  V32 : PMIOPort  Port=20  Side=Right
  V33 : PMIOPort  Port=21  Side=Right
  V34 : PMIOPort  Port=22  Side=Right
  V35 : PMIOPort  Port=23  Side=Right
  V36 : PMIOPort  Port=24  Side=Right
  V37 : PMIOPort  Port=25  Side=Right
  "V38 " : PMIOPort  Port=26  Side=Right
  Izquierda : PMIOPort  Port=27  Side=Left
  Super : PMIOPort  Port=28  Side=Left
  INFERIOR : PMIOPort  Port=29  Side=Left
  connections:
  Thermal Resistance113/RConn1 -- Thermal Mass16/LConn1 -- Thermal Resistance25/RConn1 -- Thermal Resistance118/RConn1 -- Thermal Resistance119/LConn1 -- V23/RConn1 -- Thermal Resistance137/LConn1
  Thermal Resistance143/LConn1 -- Thermal Mass14/LConn1 -- Thermal Resistance26/RConn1 -- Thermal Resistance125/RConn1 -- Thermal Resistance118/LConn1 -- V24/RConn1 -- Thermal Resistance126/LConn1
  Thermal Resistance115/LConn1 -- Thermal Resistance127/RConn1 -- Thermal Mass20/LConn1 -- Thermal Resistance33/LConn1 -- Thermal Resistance116/LConn1 -- V34/RConn1 -- Thermal Resistance126/RConn1
  Thermal Resistance129/LConn1 -- Thermal Resistance24/RConn1 -- Thermal Resistance119/RConn1 -- Thermal Mass17/LConn1 -- Thermal Resistance140/LConn1 -- V22/RConn1 -- Thermal Resistance133/LConn1
  Thermal Resistance84/RConn1 -- Thermal Resistance99/LConn1 -- V36/RConn1 -- Thermal Resistance2/LConn1 -- Thermal Mass23/LConn1 -- Thermal Resistance107/LConn1 -- Thermal Resistance102/RConn1
  Thermal Mass26/LConn1 -- Thermal Resistance1/LConn1 -- Thermal Resistance108/LConn1 -- Thermal Resistance127/LConn1 -- Thermal Resistance99/RConn1 -- Thermal Resistance100/RConn1 -- V35/RConn1
  Thermal Resistance97/LConn1 -- Thermal Resistance96/RConn1 -- Thermal Resistance86/RConn1 -- Thermal Mass22/LConn1 -- Thermal Resistance146/LConn1 -- V26/RConn1 -- Thermal Resistance102/LConn1
  Thermal Resistance80/RConn1 -- Thermal Mass5/LConn1 -- Solver Configuration/RConn1 -- Thermal Resistance85/RConn1 -- Thermal Resistance98/RConn1 -- Thermal Resistance86/LConn1 -- V27/RConn1 -- Thermal Resistance106/LConn1
  Thermal Resistance97/RConn1 -- Thermal Resistance92/RConn1 -- Thermal Mass28/LConn1 -- Thermal Resistance148/LConn1 -- V25/RConn1 -- Thermal Resistance100/LConn1 -- Thermal Resistance125/LConn1
  derecha/RConn1 -- Thermal Resistance40/LConn1 -- Thermal Resistance41/LConn1 -- Thermal Resistance39/LConn1
  Thermal Resistance15/RConn1 -- V14/RConn1 -- Thermal Resistance26/LConn1 -- Thermal Resistance27/LConn1 -- Thermal Mass4/LConn1 -- Thermal Resistance19/LConn1 -- Thermal Resistance16/RConn1
  Thermal Resistance22/RConn1 -- Thermal Mass3/LConn1 -- V13/RConn1 -- Thermal Resistance25/LConn1 -- Thermal Resistance27/RConn1 -- Thermal Resistance29/LConn1 -- Thermal Resistance18/LConn1
  Thermal Resistance28/RConn1 -- V12/RConn1 -- Thermal Resistance24/LConn1 -- Thermal Resistance29/RConn1 -- Thermal Resistance14/LConn1 -- Thermal Resistance13/LConn1 -- Thermal Mass10/LConn1
  Thermal Resistance87/RConn1 -- Thermal Mass2/LConn1 -- V17/RConn1 -- Thermal Resistance98/LConn1 -- Thermal Resistance124/RConn1 -- Thermal Resistance135/LConn1 -- Thermal Resistance74/LConn1
  Thermal Resistance73/LConn1 -- Thermal Mass30/LConn1 -- Thermal Resistance15/LConn1 -- V15/RConn1 -- Thermal Resistance92/LConn1 -- Thermal Resistance38/RConn1 -- Thermal Resistance144/RConn1
  Thermal Resistance128/RConn1 -- Thermal Mass21/LConn1 -- Thermal Resistance11/LConn1 -- V16/RConn1 -- Thermal Resistance96/LConn1 -- Thermal Resistance135/RConn1 -- Thermal Resistance38/LConn1
  Thermal Resistance22/LConn1 -- Thermal Resistance58/LConn1 -- Super/RConn1 -- Thermal Resistance87/LConn1 -- Thermal Resistance128/LConn1 -- Thermal Resistance144/LConn1 -- Thermal Resistance16/LConn1 -- Thermal Resistance59/LConn1 -- Thermal Resistance28/LConn1
  Thermal Resistance117/RConn1 -- Thermal Resistance42/LConn1 -- V32/RConn1 -- Thermal Resistance138/LConn1 -- Thermal Mass19/LConn1 -- Thermal Resistance133/RConn1 -- Thermal Resistance130/LConn1
  Thermal Resistance45/LConn1 -- Thermal Mass25/LConn1 -- Thermal Resistance117/LConn1 -- Thermal Resistance115/RConn1 -- Thermal Resistance137/RConn1 -- Thermal Resistance44/LConn1 -- V33/RConn1
  Thermal Resistance3/LConn1 -- Thermal Resistance4/LConn1 -- Thermal Mass60/LConn1 -- V37/RConn1 -- Thermal Resistance106/RConn1 -- Thermal Resistance82/RConn1 -- Thermal Resistance84/LConn1
  Thermal Resistance42/RConn1 -- Thermal Resistance57/RConn1 -- INFERIOR/RConn1 -- Thermal Resistance46/RConn1 -- Thermal Resistance4/RConn1 -- Thermal Resistance2/RConn1 -- Thermal Resistance1/RConn1 -- Thermal Resistance33/RConn1 -- Thermal Resistance44/RConn1
  Izquierda/RConn1 -- Thermal Resistance9/RConn1 -- Thermal Resistance5/RConn1 -- Thermal Resistance6/RConn1
  Thermal Resistance23/LConn1 -- Thermal Resistance5/LConn1 -- V11/RConn1 -- Thermal Resistance59/RConn1 -- Thermal Mass9/LConn1 -- Thermal Resistance17/LConn1 -- Thermal Resistance14/RConn1
  Thermal Resistance129/RConn1 -- V21/RConn1 -- Thermal Resistance23/RConn1 -- Thermal Resistance6/LConn1 -- Thermal Mass11/LConn1 -- Thermal Resistance142/LConn1 -- Thermal Resistance131/LConn1
  Thermal Resistance9/LConn1 -- Thermal Mass12/LConn1 -- V31/RConn1 -- Thermal Resistance131/RConn1 -- Thermal Resistance130/RConn1 -- Thermal Resistance139/LConn1 -- Thermal Resistance57/LConn1
  Thermal Resistance39/RConn1 -- Thermal Resistance82/LConn1 -- Thermal Mass33/LConn1 -- Thermal Resistance46/LConn1 -- Thermal Resistance308/LConn1 -- "V38 "/RConn1 -- Thermal Resistance319/RConn1
  Thermal Resistance40/RConn1 -- Thermal Resistance85/LConn1 -- Thermal Resistance145/RConn1 -- Thermal Mass27/LConn1 -- Thermal Resistance149/LConn1 -- V28/RConn1 -- Thermal Resistance319/LConn1
  Thermal Resistance145/LConn1 -- V18/RConn1 -- Thermal Resistance58/RConn1 -- Thermal Mass24/LConn1 -- Thermal Resistance76/LConn1 -- Thermal Resistance124/LConn1 -- Thermal Resistance41/RConn1
  AMB/RConn1 -- Thermal Resistance139/RConn1 -- Thermal Resistance45/RConn1 -- Thermal Resistance116/RConn1 -- Thermal Resistance108/RConn1 -- Thermal Resistance3/RConn1 -- Thermal Resistance308/RConn1 -- Thermal Resistance107/RConn1 -- Thermal Resistance138/RConn1 -- Thermal Resistance17/RConn1 -- Thermal Resistance13/RConn1 -- Thermal Resistance18/RConn1 -- Thermal Resistance73/RConn1 -- Thermal Resistance11/RConn1 -- Thermal Resistance74/RConn1 -- Thermal Resistance76/RConn1 -- Thermal Resistance19/RConn1 -- Thermal Resistance142/RConn1 -- Thermal Resistance143/RConn1 -- Thermal Resistance148/RConn1 -- Thermal Resistance149/RConn1 -- Thermal Resistance80/LConn1 -- Thermal Resistance146/RConn1 -- Thermal Resistance113/LConn1 -- Thermal Resistance140/RConn1

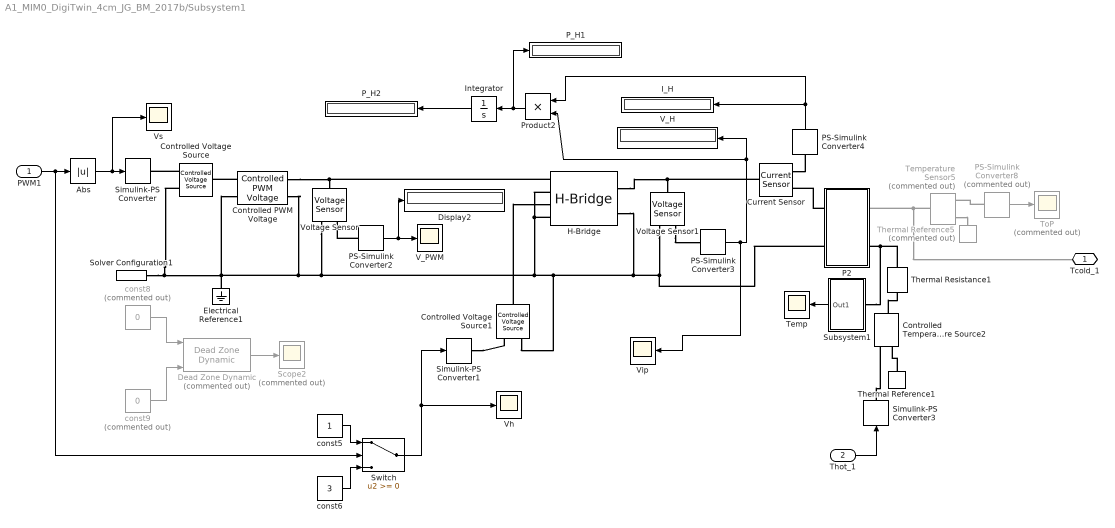
== system A1_MIM0_DigiTwin_4cm_JG_BM_2017b/Subsystem1 ==
  PWM1 : Inport
  Thot_1 : Inport  Port=2
  Abs : Abs
  Controlled Temperature Source2 : fl_lib/Thermal/Thermal Sources/Controlled Temperature Source
  Controlled PWM Voltage : ee_lib/Integrated Circuits/Controlled PWM Voltage  F=4000 Hz  TD=0 s  pulse_width_offset=0 s  pulse_min=0 s  pwm_or_av=2  event_type=1  sample_time=1e-6 s  Vmin=0 V  Vmax=5 V  Vm=5 V  u_min=0  u_max=1
  Controlled Voltage Source : fl_lib/Electrical/Electrical Sources/Controlled Voltage Source
  Controlled Voltage Source1 : fl_lib/Electrical/Electrical Sources/Controlled Voltage Source
  Current Sensor : fl_lib/Electrical/Electrical Sensors/Current Sensor
  Dead Zone Dynamic : simulink/Discontinuities/Dead Zone Dynamic  Commented=on
  Display2 : Display
  Electrical Reference1 : fl_lib/Electrical/Electrical Elements/Electrical Reference
  H-Bridge : ee_lib/Semiconductors & Converters/Converters/H-Bridge  supply_ports=ee.enum.supply_ports.hidesupply  pwm_or_av=2  regenerative_braking_mode=2  discontinuous=0  freewheeling_mode=1  Rload=10 Ohm  Lload=1e-5 H  F=10 kHz  Venable=2.5 V  Vmax=5.0 V  Vreverse=2.5 V  Vbrake=2.5 V  Vm=12 V  Ron=0.1 Ohm  Don=0.05 Ohm  Goff=1e-6 S  Tmeas=298.15 K  Ron2=0.1 Ohm  Don2=0.05 Ohm  Tmeas2=398.15 K  thermal_mass=100 J/K  initial_temperature=298.15 K
  I_H : Display
  Integrator : Integrator
  P2 : Subsystem
  PS-Simulink Converter2 : nesl_utility/PS-Simulink Converter  PhysicalDomain=network_engine_domain  SubClassName=ps_output  LeftPortType=input  RightPortType=output  PseudoPeriodic=off  Frequencies=[]  VectorFormat=1-D array  Unit=1  AffineConversion=off
  PS-Simulink Converter3 : nesl_utility/PS-Simulink Converter  PhysicalDomain=network_engine_domain  SubClassName=ps_output  LeftPortType=input  RightPortType=output  PseudoPeriodic=off  Frequencies=[]  VectorFormat=1-D array  Unit=1  AffineConversion=off
  PS-Simulink Converter4 : nesl_utility/PS-Simulink Converter  PhysicalDomain=network_engine_domain  SubClassName=ps_output  LeftPortType=input  RightPortType=output  PseudoPeriodic=off  Frequencies=[]  VectorFormat=1-D array  Unit=1  AffineConversion=off
  PS-Simulink Converter8 : nesl_utility/PS-Simulink Converter  Commented=on  PhysicalDomain=network_engine_domain  SubClassName=ps_output  LeftPortType=input  RightPortType=output  PseudoPeriodic=off  Frequencies=[]  VectorFormat=1-D array  Unit=1  AffineConversion=off
  P_H1 : Display
  P_H2 : Display
  Product2 : Product  RndMeth=Zero
  Scope2 : Scope  Commented=on
  Simulink-PS Converter : nesl_utility/Simulink-PS Converter  PhysicalDomain=network_engine_domain  SubClassName=ps_input  LeftPortType=input  RightPortType=output  PseudoPeriodic=off  Frequencies=[]  NoiseDistribution=none  NoiseParameters=[]  Unit=1  AffineConversion=off  FilteringAndDerivatives=provide  SimscapeFilterOrder=1  InputFilterTimeConstant=0.001  UdotUserProvided=0
  Simulink-PS Converter1 : nesl_utility/Simulink-PS Converter  PhysicalDomain=network_engine_domain  SubClassName=ps_input  LeftPortType=input  RightPortType=output  PseudoPeriodic=off  Frequencies=[]  NoiseDistribution=none  NoiseParameters=[]  Unit=1  AffineConversion=off  FilteringAndDerivatives=provide  SimscapeFilterOrder=1  InputFilterTimeConstant=0.001  UdotUserProvided=0
  Simulink-PS Converter3 : nesl_utility/Simulink-PS Converter  PhysicalDomain=network_engine_domain  SubClassName=ps_input  LeftPortType=input  RightPortType=output  PseudoPeriodic=off  Frequencies=[]  NoiseDistribution=none  NoiseParameters=[]  Unit=1  AffineConversion=off  FilteringAndDerivatives=provide  SimscapeFilterOrder=1  InputFilterTimeConstant=0.001  UdotUserProvided=0
  Solver Configuration1 : nesl_utility/Solver Configuration  PhysicalDomain=network_engine_domain  SubClassName=solver  LeftPortType=input  RightPortType=generic  Tones=[]  Harmonics=[]  SimulateNoise=off  Profile=off  UseLocalSampling=off  EnableSwitchedLinearOptims=on  FrequencyDomain=off  UseCCode=off  RelTol=0.001  AbsTol=1e-06  MinStep=1e-09  ToWorkspace=off  RevertToSquareIcSolve=off  NumHomotopyIterations=100  PhasorMode=off  PhasorModeNumHarmonics=1  ConsistencySolver=NEWTON_FTOL  IndexReductionMethod=DerivativeReplacement  DoDC=off  ResidualTolerance=1e-09  ConsistencyTolSource=GLOBAL  ConsistencyAbsTol=0.001  ConsistencyRelTol=0.001  ConsistencyTolFactor=0.001  UseLocalSolver=off  LocalSolverChoice=NE_BACKWARD_EULER_ADVANCER  ResolveIndetEquations=on  FunctionEvalNumThread=1  LocalSolverSampleTime=0.001  DoFixedCost=off  MaxNonlinIter=3  MaxModeIter=2  ComputeImpulses=off  ImpulseIterations=2  LinearAlgebra=Sparse  LinearAlgebraNumThread=0  EquationFormulation=NE_TIME_EF  DelaysMemoryBudget=1024  AutomaticFiltering=on  FilteringTimeConstant=0.001  PartitionStorageMethod=AS_NEEDED  PartitionMemoryBudget=1024  PartitionMethod=FAST
  Subsystem1 : Subsystem
  Switch : Switch
  Temp : Scope
  Temperature Sensor5 : fl_lib/Thermal/Thermal Sensors/Temperature Sensor  Commented=on
  Thermal Reference1 : fl_lib/Thermal/Thermal Elements/Thermal Reference
  Thermal Reference5 : fl_lib/Thermal/Thermal Elements/Thermal Reference  Commented=on
  Thermal Resistance1 : fl_lib/Thermal/Thermal Elements/Thermal Resistance  resistance=Rph K/W  T_specify=off  T_priority=None  T=0 K  T_nominal_specify=off  T_nominal_unit=K  T_nominal_value=1  Q_specify=off  Q_priority=None  Q=0 W  Q_nominal_specify=off  Q_nominal_unit=W  Q_nominal_value=1
  ToP : Scope  Commented=on
  V_H : Display
  V_PWM : Scope
  Vh : Scope
  Vip : Scope
  Voltage Sensor : fl_lib/Electrical/Electrical Sensors/Voltage Sensor
  Voltage Sensor1 : fl_lib/Electrical/Electrical Sensors/Voltage Sensor
  Vs : Scope
  const5 : Constant
  const6 : Constant  Value=3
  const8 : Constant  Commented=on  Value=0
  const9 : Constant  Commented=on  Value=0
  Tcold_1 : PMIOPort  Side=Right
  wires:
  Switch/1 -> Simulink-PS Converter1/1, Vh/1
  PS-Simulink Converter8/1 -> ToP/1
  PS-Simulink Converter2/1 -> Display2/1, V_PWM/1
  Subsystem1/1(Out1) -> Temp/1
  Thot_1/1 -> Simulink-PS Converter3/1
  const5/1 -> Switch/1
  PWM1/1 -> Switch/2, Abs/1
  const6/1 -> Switch/3
  Abs/1 -> Vs/1, Simulink-PS Converter/1
  Integrator/1 -> P_H2/1
  PS-Simulink Converter4/1 -> Product2/1, I_H/1
  PS-Simulink Converter3/1 -> Vip/1, Product2/2, V_H/1
  Product2/1 -> P_H1/1, Integrator/1
  const9/1 -> Dead Zone Dynamic/3
  Dead Zone Dynamic/1 -> Scope2/1
  const8/1 -> Dead Zone Dynamic/1
  connections:
  Temperature Sensor5/RConn1 -- Thermal Reference5/LConn1
  Simulink-PS Converter1/RConn1 -- Controlled Voltage Source1/RConn1
  P2/LConn1 -- Current Sensor/RConn2
  Controlled PWM Voltage/LConn1 -- Controlled Voltage Source/LConn1
  Controlled Voltage Source1/LConn1 -- H-Bridge/LConn3
  PS-Simulink Converter8/LConn1 -- Temperature Sensor5/RConn2
  Voltage Sensor1/RConn1 -- PS-Simulink Converter3/LConn1
  Controlled PWM Voltage/RConn1 -- H-Bridge/LConn1 -- Voltage Sensor/LConn1
  Controlled Voltage Source/RConn1 -- Simulink-PS Converter/RConn1
  Temperature Sensor5/LConn1 -- Tcold_1/RConn1 -- P2/RConn1
  PS-Simulink Converter2/LConn1 -- Voltage Sensor/RConn1
  H-Bridge/RConn1 -- Current Sensor/LConn1 -- Voltage Sensor1/LConn1
  Current Sensor/RConn1 -- PS-Simulink Converter4/LConn1
  Thermal Resistance1/RConn1 -- Subsystem1/LConn1 -- P2/RConn2
  Simulink-PS Converter3/RConn1 -- Controlled Temperature Source2/RConn1
  Thermal Reference1/LConn1 -- Controlled Temperature Source2/RConn2
  Controlled Temperature Source2/LConn1 -- Thermal Resistance1/LConn1
  Electrical Reference1/LConn1 -- Controlled Voltage Source/RConn2 -- Solver Configuration1/RConn1 -- H-Bridge/LConn4 -- H-Bridge/LConn2 -- Controlled Voltage Source1/RConn2 -- P2/LConn2 -- Voltage Sensor1/RConn2 -- H-Bridge/RConn2 -- Voltage Sensor/RConn2 -- Controlled PWM Voltage/RConn2 -- Controlled PWM Voltage/LConn2

== system A1_MIM0_DigiTwin_4cm_JG_BM_2017b/Subsystem10 ==
  PS-Simulink Converter1 : nesl_utility/PS-Simulink Converter  PhysicalDomain=network_engine_domain  SubClassName=ps_output  LeftPortType=input  RightPortType=output  PseudoPeriodic=off  Frequencies=[]  VectorFormat=1-D array  Unit=1  AffineConversion=off
  Temperature Sensor2 : fl_lib/Thermal/Thermal Sensors/Temperature Sensor
  Thermal Reference4 : fl_lib/Thermal/Thermal Elements/Thermal Reference
  Conn1 : PMIOPort  Side=Left
  Out1 : Outport  VectorParamsAs1DForOutWhenUnconnected=off
  wires:
  PS-Simulink Converter1/1 -> Out1/1
  connections:
  Temperature Sensor2/LConn1 -- Conn1/RConn1
  PS-Simulink Converter1/LConn1 -- Temperature Sensor2/RConn2
  Thermal Reference4/LConn1 -- Temperature Sensor2/RConn1

== system A1_MIM0_DigiTwin_4cm_JG_BM_2017b/Subsystem2 ==
  PS-Simulink Converter1 : nesl_utility/PS-Simulink Converter  PhysicalDomain=network_engine_domain  SubClassName=ps_output  LeftPortType=input  RightPortType=output  PseudoPeriodic=off  Frequencies=[]  VectorFormat=1-D array  Unit=1  AffineConversion=off
  PS-Simulink Converter5 : nesl_utility/PS-Simulink Converter  PhysicalDomain=network_engine_domain  SubClassName=ps_output  LeftPortType=input  RightPortType=output  PseudoPeriodic=off  Frequencies=[]  VectorFormat=1-D array  Unit=1  AffineConversion=off
  Temperature Sensor1 : fl_lib/Thermal/Thermal Sensors/Temperature Sensor
  Temperature Sensor5 : fl_lib/Thermal/Thermal Sensors/Temperature Sensor
  Thermal Reference1 : fl_lib/Thermal/Thermal Elements/Thermal Reference
  Thermal Reference5 : fl_lib/Thermal/Thermal Elements/Thermal Reference
  To Workspace1 : ToWorkspace  VariableName=Tair  SampleTime=-1
  To Workspace5 : ToWorkspace  VariableName=Tais  SampleTime=-1
  TemAis1 : PMIOPort  Side=Left
  TemAir2 : PMIOPort  Port=2  Side=Left
  O1 : Outport  VectorParamsAs1DForOutWhenUnconnected=off
  O2 : Outport  Port=2  VectorParamsAs1DForOutWhenUnconnected=off
  wires:
  PS-Simulink Converter5/1 -> To Workspace5/1, O1/1
  PS-Simulink Converter1/1 -> To Workspace1/1, O2/1
  connections:
  Temperature Sensor5/RConn1 -- Thermal Reference5/LConn1
  PS-Simulink Converter5/LConn1 -- Temperature Sensor5/RConn2
  PS-Simulink Converter1/LConn1 -- Temperature Sensor1/RConn2
  Temperature Sensor1/RConn1 -- Thermal Reference1/LConn1
  Temperature Sensor5/LConn1 -- TemAis1/RConn1
  Temperature Sensor1/LConn1 -- TemAir2/RConn1
